simulink model "HW1_2"  (R2025b)
settings: Solver=VariableStepAuto  StartTime=0.0  StopTime=20  RelTol=1e-3
libraries: simulink x1
settings Model: Creator=yunzhuorui  LastModifiedBy=yunzhuorui

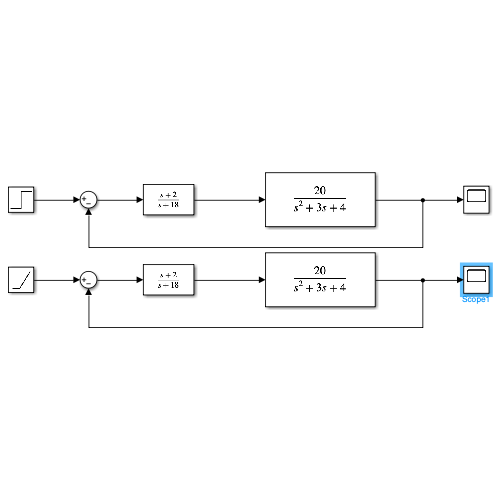
[thumbnail: Simulink's stored preview of the top-level diagram]
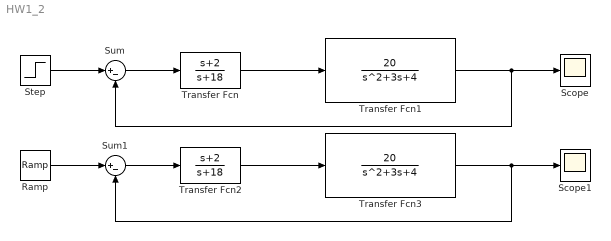
== system HW1_2 ==
  Ramp : simulink/Sources/Ramp  slope=5  start=0  InitialOutput=0
  Scope : Scope
      settings: ActiveDisplayYMinimum=-0.26089136088196324  ActiveDisplayYMaximum=2.34802224793767
  Scope1 : Scope
      settings: ActiveDisplayYMinimum=-4.4204400505890371  ActiveDisplayYMaximum=39.78396045530134
  Step : Step  After=5  SampleTime=0
  Sum : Sum  Inputs=|+-
  Sum1 : Sum  Inputs=|+-
  Transfer Fcn : TransferFcn  Numerator=[1 2]  Denominator=[1 18]
  Transfer Fcn1 : TransferFcn  Numerator=[20]  Denominator=[1 3 4]
  Transfer Fcn2 : TransferFcn  Numerator=[1 2]  Denominator=[1 18]
  Transfer Fcn3 : TransferFcn  Numerator=[20]  Denominator=[1 3 4]
  wires:
  Step/1 -> Sum/1
  Sum/1 -> Transfer Fcn/1
  Transfer Fcn/1 -> Transfer Fcn1/1
  Transfer Fcn1/1 -> Sum/2, Scope/1
  Transfer Fcn2/1 -> Transfer Fcn3/1
  Sum1/1 -> Transfer Fcn2/1
  Transfer Fcn3/1 -> Sum1/2, Scope1/1
  Ramp/1 -> Sum1/1
